simulink model "fcsystemBechmarkold"  (R2016a)
settings: Solver=FixedStepAuto  SolverMode=MultiTasking  StartTime=0.0  StopTime=30.0  FixedStep=0.0001  MaxStep=0.0001  RelTol=1e-5
InitFcn:
  | fcsmain;
values from neighbouring files (symbols this model uses):
  C = ss1.C    [MVE.m]
  G = ss1.A    [MVE.m]
  H = ss1.B    [MVE.m]
  K1 = Ktemp(1)    [MVE.m]
  K2 = Ktemp(2:end)    [MVE.m]
  Ke = acker(G',C',P)'    [MVE.m]
  Ts = 0.1    [MVE.m]
undefined symbols (not defined in the file or in its folder): alliedsignaleff, beta0, beta1, beta2, cm_kt, cm_kv, cm_maxtorque, cm_R, Cp, cp_inertia, dc, faradays, fc_activearea, fc_anode_volume, fc_cathode_volume, fc_inlet_flow_constant, fc_numberofcells, fc_outlet_flow_constant, fcx0, gamma, hydrogengasconstant, hydrogenmolarmass, im_volume, membranedrydensity, membranedryeqvweight, membranethickness, nitrogengasconstant, nitrogenmolarmass, om_At, om_Cd, om_outlet_choke_pr, om_volume, oxygengasconstant, oxygenmolarmass, phimax0, phimax1, phimax2, phimax3, phimax4, psimax0, psimax1, psimax2, psimax3, psimax4, psimax5, R, rho, Ta, universalgasconstant, vaporgasconstant, vapormolarmass
libraries: simulink x1
(part 1 of 3)
settings Model: ExtModeTrigMode=oneshot  ExtModeArmWhenConnect=off  Creator=Jay Tawee Pukrushpan  LastModifiedBy=luisd
settings DataIOCC: SaveFinalState=on  SaveFormat=Array  SignalLoggingSaveFormat=ModelDataLogs  SignalLoggingName=sigsOut
settings OptimizationCC: BooleanDataType=off
settings DebuggingCC: SaveWithParameterizedLinksMsg=none  UnderspecifiedInitializationDetection=Classic  MergeDetectMultiDrivingBlocksExec=none  SignalResolutionControl=TryResolveAllWithWarning  MultiTaskDSMMsg=warning  MultiTaskCondExecSysMsg=none  FcnCallInpInsideContextMsg=UseLocalSettings  AllowSymbolicDim=off  StateNameClashWarn=warning
settings HardwareCC: ProdBitPerPointer=32  ProdLargestAtomicFloat=None  ProdIntDivRoundTo=Undefined  ProdEndianess=Unspecified  ProdWordSize=32  ProdHWDeviceType=32-bit Generic  TargetUnknown=on
settings ModelReferenceCC: PropagateSignalLabelsOutOfModel=off
settings GRTTargetCC: CombineOutputUpdateFcns=off  GRTInterface=on
settings ConfigComp: CovModelRefEnable=Off  CovSFcnEnable=off

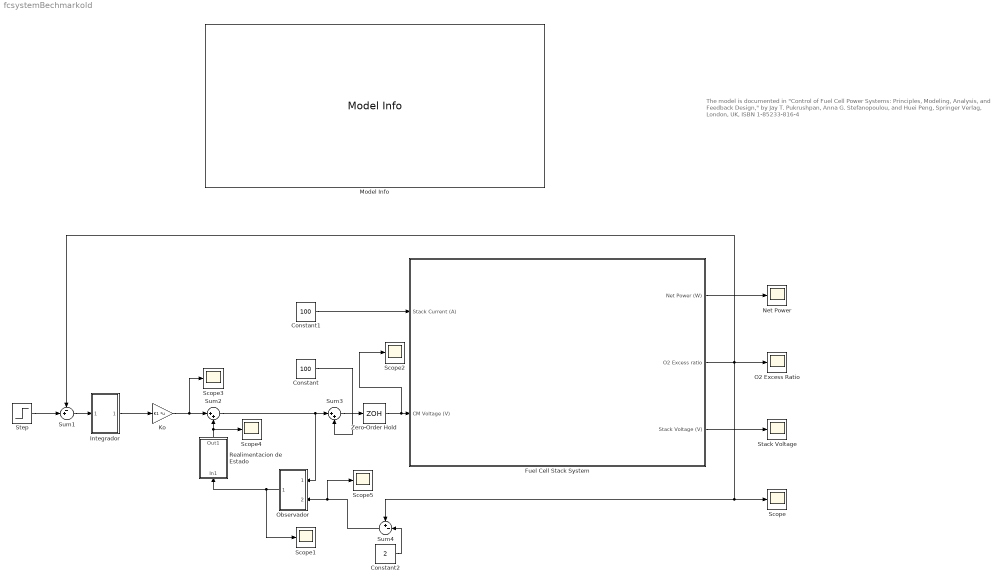
== system fcsystemBechmarkold ==
  note: The model is documented in
      | "Control of Fuel Cell Power Systems: Principles, Modeling, Analysis, and Feedback Design,"
      | by  Jay T. Pukrushpan, Anna G. Stefanopoulou, and Huei Peng,  Springer Verlag,
      | London, UK, ISBN 1-85233-816-4
  Constant : Constant  Value=100
  Constant1 : Constant  Value=100
  Constant2 : Constant  Value=2
  Fuel Cell Stack System : Subsystem
      mask Display:
      | image('Stack.jpg')
      | port_label('input', 1, 'corriente carga')
      | port_label('input', 2, 'tension compresor')
      | port_label('output', 1, 'potencia salida')
      | port_label('output', 2, 'exceso de oxigeno')
      | port_label('output', 3, 'tension de la pila')
  Integrador : Subsystem
  Ko : Gain  Gain=K1  Multiplication=Matrix(K*u)
  Model Info : simulink/Model-Wide Utilities/Model Info  Frame=on  DisplayStringWithTags=|  HorizontalTextAlignment=Left  LeftAlignmentValue=0.02  SourceBlockDiagram=fcsystemBechmark  TagMaxNumber=20
      | COPYRIGHT  © 2002 
      | THE REGENTS OF THE UNIVERSITY OF MICHIGAN
      | ALL RIGHTS RESERVED
      |       
      | PERMISSION IS GRANTED TO USE, COPY, CREATE DERIVATIVE WORKS AND REDISTRIBUTE THIS SOFTWARE AND SUCH 
      | DERIVATIVE WORKS FOR NONCOMMERCIAL EDUCATION AND RESEARCH PURPOSES, SO LONG AS NO FEE IS CHARGED, AND 
      | SO LONG AS THE COPYRIGHT NOTICE ABOVE, THIS GRANT OF PERMISSION, AND THE DISCLAIMER BELOW APPEAR IN ALL 
      | COPIES MADE; AND SO LONG AS THE NAME OF THE UNIVERSITY OF MICHIGAN IS NOT USED IN ANY ADVERTISING OR PUBLICITY 
      | PERTAINING TO THE USE OR DISTRIBUTION OF THIS SOFTWARE WITHOUT SPECIFIC, WRITTEN PRIOR AUTHORIZATION.
      |     
      | THIS USE OF THIS SOFTWARE REQUIRES SIMULINK, A LICENSED PRODUCT OF THE MATHWORKS, INC.  THE SOFTWARE 
      | USER IS SOLELY RESOPNSIBLE FOR OBTAINTING AN APPROPRIATE LICENSE FOR SIMULINK.  NO LICENSE TO SIMULINK 
      | IS GRANTED, INFERRED OR IMPLIED BY THE DISTRIBUTION OF THIS SOFTWARE.
      |     
      | THIS SOFTWARE IS PROVIDED AS IS, WITHOUT REPRESENTATION AS TO ITS FITNESS FOR ANY PURPOSE, AND WITHOUT 
      | WARRANTY OF ANY KIND, EITHER EXPRESS OR IMPLIED, INCLUDING WITHOUT LIMITATION THE IMPLIED WARRANTIES OF 
      | MERCHANTABILITY AND FITNESS FOR A PARTICULAR PURPOSE. THE REGENTS OF THE UNIVERSITY OF MICHIGAN SHALL NOT 
      | BE LIABLE FOR ANY DAMAGES, INCLUDING SPECIAL, INDIRECT, INCIDENTAL, OR CONSEQUENTIAL DAMAGES, WITH RESPECT
      | TO ANY CLAIM ARISING OUT OF OR IN CONNECTION WITH THE USE OF THE SOFTWARE, EVEN IF IT HAS BEEN OR IS HEREAFTER 
      | ADVISED OF THE POSSIBILITY OF SUCH DAMAGES.
  Net Power : Scope
  O2 Excess Ratio : Scope
  Observador : Subsystem
  Realimentacion de Estado : Subsystem
  Scope{,1..5} (6 alike) : Scope
  Stack Voltage : Scope
  Step : Step  Time=0  Before=2  After=2  SampleTime=Ts
  Sum1 : Sum  Inputs=-+|
  Sum2 : Sum  Inputs=|++
  Sum3 : Sum  Inputs=|++
  Sum4 : Sum  Inputs=+-|
  Zero-Order Hold : ZeroOrderHold  SampleTime=Ts
  wires:
  Sum2/1 -> Sum3/1, Observador/1(In1)
  Fuel Cell Stack System/1(Net Power (W)) -> Net Power/1
  Fuel Cell Stack System/3(Stack Voltage (V)) -> Stack Voltage/1
  Ko/1 -> Scope3/1, Sum2/1
  Realimentacion de Estado/1(Out1) -> Scope4/1, Sum2/2
  Observador/1(Out1) -> Scope1/1, Realimentacion de Estado/1(In1)
  Integrador/1(Out1) -> Ko/1
  Sum1/1 -> Integrador/1(In1)
  Step/1 -> Sum1/2
  Fuel Cell Stack System/2(O2 Excess ratio) -> Sum1/1, Sum4/1, Scope/1, O2 Excess Ratio/1
  Zero-Order Hold/1 -> Scope2/1, Fuel Cell Stack System/2(CM Voltage (V))
  Sum3/1 -> Zero-Order Hold/1
  Constant/1 -> Sum3/2
  Constant2/1 -> Sum4/2
  Sum4/1 -> Scope5/1, Observador/2(In2)
  Constant1/1 -> Fuel Cell Stack System/1(Stack Current (A))

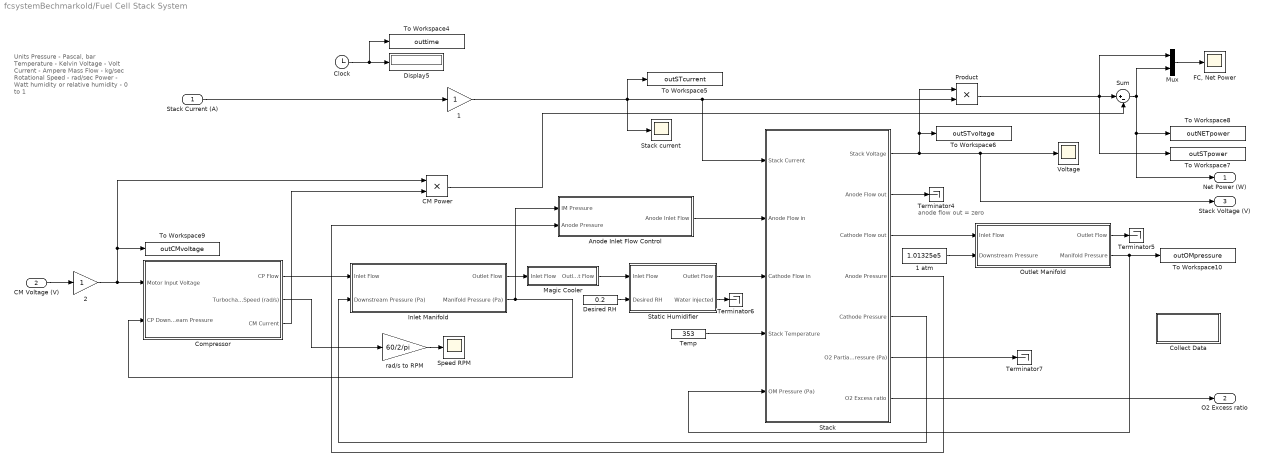
== system fcsystemBechmarkold/Fuel Cell Stack System ==
  note: Units
      | Pressure - Pascal, bar
      | Temperature - Kelvin
      | Voltage - Volt
      | Current - Ampere
      | Mass Flow - kg/sec
      | Rotational Speed - rad/sec
      | Power - Watt
      | humidity or relative humidity - 0 to 1
  note: anode flow out = zero
  Stack Current (A) : Inport
  CM Voltage (V) : Inport  Port=2
  " Outlet Manifold" : Subsystem
  1 : Gain  SaturateOnIntegerOverflow=on  OutDataTypeStr=Inherit: Same as input  ParamDataTypeStr=Inherit: Same as input
  1 atm : Constant  Value=1.01325e5
  2 : Gain  SaturateOnIntegerOverflow=on  OutDataTypeStr=Inherit: Same as input  ParamDataTypeStr=Inherit: Same as input
  Anode Inlet Flow Control : Subsystem
  CM Power : Product  SaturateOnIntegerOverflow=on  InputSameDT=on  OutDataTypeStr=Inherit: Same as first input
  Clock : Clock
  Collect Data : Subsystem
  Compressor : Subsystem
  Desired RH : Constant  Value=0.2
  Display5 : Display
  "FC, Net Power" : Scope
  Inlet Manifold : Subsystem
  Magic Cooler : Subsystem
  Mux : Mux  Inputs=2
  Product : Product  SaturateOnIntegerOverflow=on  InputSameDT=on  OutDataTypeStr=Inherit: Same as first input
  Speed RPM : Scope
  Stack : Subsystem
  Stack current : Scope
  Static Humidifier : Subsystem
  Sum : Sum  Inputs=|+-  SaturateOnIntegerOverflow=on  InputSameDT=on  OutDataTypeStr=Inherit: Same as first input
  Temp : Constant  Value=353
  Terminator{4..7} (4 alike) : Terminator
  To Workspace10 : ToWorkspace  VariableName=outOMpressure  SampleTime=-1
  To Workspace4 : ToWorkspace  VariableName=outtime  SampleTime=-1
  To Workspace5 : ToWorkspace  VariableName=outSTcurrent  SampleTime=-1
  To Workspace6 : ToWorkspace  VariableName=outSTvoltage  SampleTime=-1
  To Workspace7 : ToWorkspace  VariableName=outSTpower  SampleTime=-1
  To Workspace8 : ToWorkspace  VariableName=outNETpower  SampleTime=-1
  To Workspace9 : ToWorkspace  VariableName=outCMvoltage  SampleTime=-1
  Voltage : Scope
  rad/s to RPM : Gain  Gain=60/2/pi  SaturateOnIntegerOverflow=on  OutDataTypeStr=Inherit: Same as input  ParamDataTypeStr=Inherit: Same as input
  Net Power (W) : Outport
  O2 Excess ratio : Outport  Port=2
  Stack Voltage (V) : Outport  Port=3
  wires:
  Temp/1 -> Stack/4(Stack Temperature)
  Anode Inlet Flow Control/1(Anode Inlet Flow) -> Stack/2(Anode Flow in)
  rad/s to RPM/1 -> Speed RPM/1
  Inlet Manifold/1(Outlet Flow) -> Magic Cooler/1(Inlet Flow)
  1/1 -> Stack/1(Stack Current), Product/2, To Workspace5/1, Stack current/1
  Compressor/1(CP Flow) -> Inlet Manifold/1(Inlet Flow)
  Compressor/2(Turbocharger Speed (rad/s)) -> rad/s to RPM/1
  Magic Cooler/1(Outlet Flow) -> Static Humidifier/1(Inlet Flow)
  Desired RH/1 -> Static Humidifier/2(Desired RH)
  Stack/2(Anode Flow out) -> Terminator4/1
  " Outlet Manifold"/1(Outlet Flow) -> Terminator5/1
  Stack/4(Anode Pressure) -> Anode Inlet Flow Control/2(Anode Pressure)
  Product/1 -> To Workspace7/1, Mux/1, Sum/1
  Mux/1 -> "FC, Net Power"/1
  Sum/1 -> Mux/2, To Workspace8/1, Net Power (W)/1
  Stack/3(Cathode Flow out) -> " Outlet Manifold"/1(Inlet Flow)
  1 atm/1 -> " Outlet Manifold"/2(Downstream Pressure)
  " Outlet Manifold"/2(Manifold Pressure) -> To Workspace10/1, Stack/5(OM Pressure (Pa))
  Static Humidifier/2(Water injected) -> Terminator6/1
  Static Humidifier/1(Outlet Flow) -> Stack/3(Cathode Flow in)
  CM Power/1 -> Sum/2
  Clock/1 -> To Workspace4/1, Display5/1
  Compressor/3(CM Current) -> CM Power/2
  Stack/5(Cathode Pressure) -> Inlet Manifold/2(Downstream Pressure (Pa))
  Inlet Manifold/2(Manifold Pressure (Pa)) -> Anode Inlet Flow Control/1(IM Pressure), Compressor/2(CP Downstream Pressure)
  Stack/6(O2 Partial Pressure (Pa)) -> Terminator7/1
  CM Voltage (V)/1 -> 2/1
  Stack/7(O2 Excess ratio) -> O2 Excess ratio/1
  Stack/1(Stack Voltage) -> Product/1, To Workspace6/1, Stack Voltage (V)/1, Voltage/1
  2/1 -> Compressor/1(Motor Input Voltage), To Workspace9/1, CM Power/1
  Stack Current (A)/1 -> 1/1

== system fcsystemBechmarkold/Integrador ==
  In1 : Inport
  Delay : Delay  DelayLength=1  InitialCondition=0  SampleTime=Ts
  Sum1 : Sum  Inputs=|++
  Out1 : Outport
  wires:
  Sum1/1 -> Out1/1, Delay/1
  In1/1 -> Sum1/1
  Delay/1 -> Sum1/2

== system fcsystemBechmarkold/Observador ==
  In1 : Inport
  In2 : Inport  Port=2
  C : Gain  Gain=C  Multiplication=Matrix(K*u)
  Delay : Delay  DelayLength=1  InitialCondition=1  SampleTime=Ts
  G : Gain  Gain=G  Multiplication=Matrix(K*u)
  H : Gain  Gain=H  Multiplication=Matrix(K*u)
  Ke : Gain  Gain=Ke  Multiplication=Matrix(K*u)
  Sum1 : Sum  Inputs=-+|
  Sum3 : Sum  Inputs=|++
  Sum4 : Sum  Inputs=|++
  Out1 : Outport
  wires:
  In2/1 -> Sum1/2
  Ke/1 -> Sum4/2
  G/1 -> Sum3/2
  C/1 -> Sum1/1
  Delay/1 -> Out1/1, G/1, C/1
  Sum4/1 -> Sum3/1
  In1/1 -> H/1
  Sum3/1 -> Delay/1
  H/1 -> Sum4/1
  Sum1/1 -> Ke/1

== system fcsystemBechmarkold/Realimentacion de Estado ==
  In1 : Inport
  K : Gain  Gain=-K2  Multiplication=Matrix(K*u)
  Out1 : Outport
  wires:
  K/1 -> Out1/1
  In1/1 -> K/1

== system fcsystemBechmarkold/Fuel Cell Stack System/ Outlet Manifold ==
  Inlet Flow : Inport
  Downstream Pressure : Inport  Port=2
  1 - Total Mass Flow 2 - Temperature 3 - Pressure 4 - Relative Humidity 5 - Oxygen Mole Fraction (in Dry Air) : Demux  Outputs=5
  1 - Total Mass Flow 2 - Temperature 3 - Pressure 4 - Relative Humidity 5 - Oxygen Mole Fraction (in Dry Air)1 : Mux  Inputs=5
  Gain1 : Gain  Gain=R  SaturateOnIntegerOverflow=on  OutDataTypeStr=Inherit: Same as input  ParamDataTypeStr=Inherit: Same as input
  Gain2 : Gain  Gain=1/om_volume  SaturateOnIntegerOverflow=on  OutDataTypeStr=Inherit: Same as input  ParamDataTypeStr=Inherit: Same as input
  Initial P_om : Constant  Value=fcx0(8)
  Nonlinear Nozzle : Subsystem
  P_om Integrator : Integrator  InitialConditionSource=external
  Product : Product  SaturateOnIntegerOverflow=on  InputSameDT=on  OutDataTypeStr=Inherit: Same as first input
  Sum1 : Sum  Inputs=|+-  SaturateOnIntegerOverflow=on  InputSameDT=on  OutDataTypeStr=Inherit: Same as first input
  Terminator7 : Terminator
  Outlet Flow : Outport
  Manifold Pressure : Outport  Port=2
  tag scope: P_om=global
  wires:
  Downstream Pressure/1 -> Nonlinear Nozzle/2(Atmospheric Pressure)
  1 - Total Mass Flow 2 - Temperature 3 - Pressure 4 - Relative Humidity 5 - Oxygen Mole Fraction (in Dry Air)/5 -> 1 - Total Mass Flow 2 - Temperature 3 - Pressure 4 - Relative Humidity 5 - Oxygen Mole Fraction (in Dry Air)1/5
  1 - Total Mass Flow 2 - Temperature 3 - Pressure 4 - Relative Humidity 5 - Oxygen Mole Fraction (in Dry Air)/4 -> 1 - Total Mass Flow 2 - Temperature 3 - Pressure 4 - Relative Humidity 5 - Oxygen Mole Fraction (in Dry Air)1/4
  Nonlinear Nozzle/1(Mass Air Flow) -> 1 - Total Mass Flow 2 - Temperature 3 - Pressure 4 - Relative Humidity 5 - Oxygen Mole Fraction (in Dry Air)1/1, Sum1/2
  1 - Total Mass Flow 2 - Temperature 3 - Pressure 4 - Relative Humidity 5 - Oxygen Mole Fraction (in Dry Air)1/1 -> Outlet Flow/1
  1 - Total Mass Flow 2 - Temperature 3 - Pressure 4 - Relative Humidity 5 - Oxygen Mole Fraction (in Dry Air)/3 -> Terminator7/1
  1 - Total Mass Flow 2 - Temperature 3 - Pressure 4 - Relative Humidity 5 - Oxygen Mole Fraction (in Dry Air)/1 -> Sum1/1
  Inlet Flow/1 -> 1 - Total Mass Flow 2 - Temperature 3 - Pressure 4 - Relative Humidity 5 - Oxygen Mole Fraction (in Dry Air)/1
  1 - Total Mass Flow 2 - Temperature 3 - Pressure 4 - Relative Humidity 5 - Oxygen Mole Fraction (in Dry Air)/2 -> 1 - Total Mass Flow 2 - Temperature 3 - Pressure 4 - Relative Humidity 5 - Oxygen Mole Fraction (in Dry Air)1/2, Nonlinear Nozzle/3(Flow Temp), Gain1/1
  Gain1/1 -> Gain2/1
  Sum1/1 -> Product/1
  Gain2/1 -> Product/2
  P_om Integrator/1 -> 1 - Total Mass Flow 2 - Temperature 3 - Pressure 4 - Relative Humidity 5 - Oxygen Mole Fraction (in Dry Air)1/3, Manifold Pressure/1, [P_om], Nonlinear Nozzle/1(Manifold Pressure)
  Product/1 -> P_om Integrator/1
  Initial P_om/1 -> P_om Integrator/2

== system fcsystemBechmarkold/Fuel Cell Stack System/Anode Inlet Flow Control ==
  IM Pressure : Inport
  Anode Pressure : Inport  Port=2
  1 - Total Mass Flow 2 - Temperature 3 - Pressure 4 - Relative Humidity : Mux
  Gain : Gain  SaturateOnIntegerOverflow=on  OutDataTypeStr=Inherit: Same as input  ParamDataTypeStr=Inherit: Same as input
  Gain1 : Gain  Gain=2.1e-6  SaturateOnIntegerOverflow=on  OutDataTypeStr=Inherit: Same as input  ParamDataTypeStr=Inherit: Same as input
  RH : Constant  Value=0.4
  Sum : Sum  Inputs=|+-  SaturateOnIntegerOverflow=on  InputSameDT=on  OutDataTypeStr=Inherit: Same as first input
  Temp : Constant  Value=353
  pim to pca map : Fcn  Expr=(0.00092256030284*u+2.84870103138421)*1e3
  Anode Inlet Flow : Outport
  wires:
  Anode Pressure/1 -> 1 - Total Mass Flow 2 - Temperature 3 - Pressure 4 - Relative Humidity/3, Sum/2
  pim to pca map/1 -> Sum/1
  IM Pressure/1 -> pim to pca map/1
  Gain1/1 -> Gain/1
  Sum/1 -> Gain1/1
  RH/1 -> 1 - Total Mass Flow 2 - Temperature 3 - Pressure 4 - Relative Humidity/4
  Gain/1 -> 1 - Total Mass Flow 2 - Temperature 3 - Pressure 4 - Relative Humidity/1
  Temp/1 -> 1 - Total Mass Flow 2 - Temperature 3 - Pressure 4 - Relative Humidity/2
  1 - Total Mass Flow 2 - Temperature 3 - Pressure 4 - Relative Humidity/1 -> Anode Inlet Flow/1

== system fcsystemBechmarkold/Fuel Cell Stack System/Collect Data ==
  Mux : Mux  Inputs=9
  To Workspace : ToWorkspace  VariableName=outstates  SampleTime=-1
  wires:
  Mux/1 -> To Workspace/1
  [mw_ca] -> Mux/9
  [P_om] -> Mux/8
  [mw_an] -> Mux/7
  [m_im] -> Mux/6
  [P_im] -> Mux/5
  [w_cp] -> Mux/4
  [mN2] -> Mux/3
  [mH2] -> Mux/2
  [mO2] -> Mux/1

== system fcsystemBechmarkold/Fuel Cell Stack System/Compressor ==
  Motor Input Voltage : Inport
  CP Downstream Pressure : Inport  Port=2
  Compressor : Subsystem
  Constant : Constant  Value=0
  Constant1 : Constant  Value=0.5
  Static Motor : Subsystem
  To Workspace1 : ToWorkspace  VariableName=outCPspeed  SampleTime=-1
  To Workspace3 : ToWorkspace  VariableName=outCPpower  SampleTime=-1
  To Workspace4 : ToWorkspace  VariableName=outCMpower  SampleTime=-1
  Turbocharger Inertia : Subsystem
  CP Flow : Outport
  Turbocharger Speed (rad/s) : Outport  Port=2
  CM Current : Outport  Port=3
  wires:
  Static Motor/2(Motor Current) -> CM Current/1
  Motor Input Voltage/1 -> Static Motor/1(Input Voltage)
  Static Motor/1(Motor Power) -> To Workspace4/1, Turbocharger Inertia/1(Motor Power)
  Compressor/2(Power) -> To Workspace3/1, Turbocharger Inertia/2(Compressor Power)
  Constant1/1 -> Compressor/3(Inlet Humidity)
  Turbocharger Inertia/1(Speed) -> To Workspace1/1, Turbocharger Speed (rad/s)/1, Compressor/2(Speed), Static Motor/2(Motor Speed (rad/s))
  CP Downstream Pressure/1 -> Compressor/1(Exit Pressure (Pa))
  Compressor/1(CP Flow) -> CP Flow/1
  Constant/1 -> Turbocharger Inertia/3(Turbine Power)

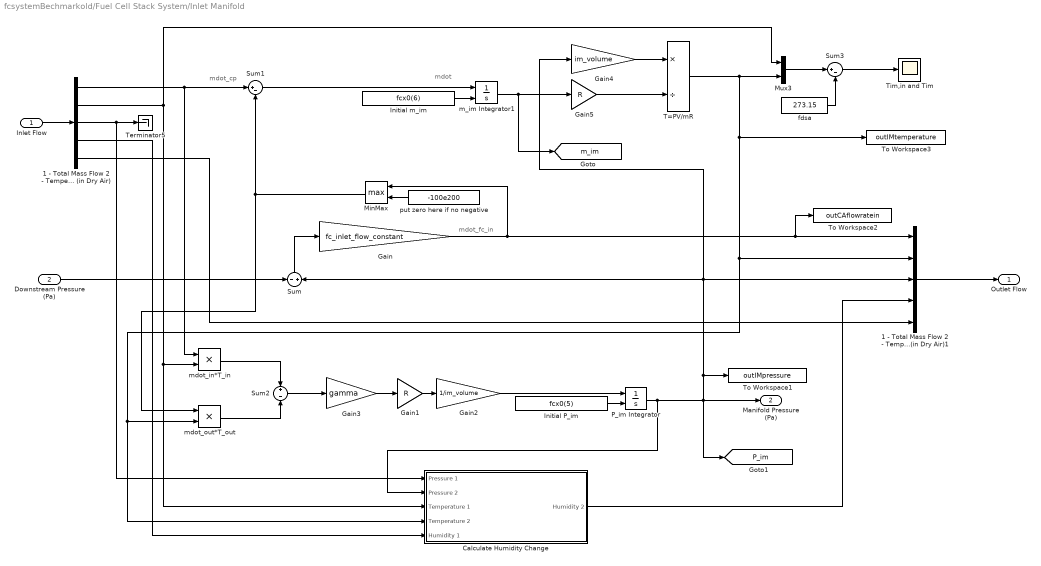
== system fcsystemBechmarkold/Fuel Cell Stack System/Inlet Manifold ==
  note: mdot_cp
  note: mdot_fc_in
  note: mdot
  Inlet Flow : Inport
  Downstream Pressure (Pa) : Inport  Port=2
  1 - Total Mass Flow 2 - Temperature 3 - Pressure 4 - Relative Humidity 5 - Oxygen Mole Fraction (in Dry Air) : Demux  Outputs=5
  1 - Total Mass Flow 2 - Temperature 3 - Pressure 4 - Relative Humidity 5 - Oxygen Mole Fraction (in Dry Air)1 : Mux  Inputs=5
  Calculate Humidity Change : Subsystem
  Gain : Gain  Gain=fc_inlet_flow_constant  SaturateOnIntegerOverflow=on  OutDataTypeStr=Inherit: Same as input  ParamDataTypeStr=Inherit: Same as input
  Gain1 : Gain  Gain=R  SaturateOnIntegerOverflow=on  OutDataTypeStr=Inherit: Same as input  ParamDataTypeStr=Inherit: Same as input
  Gain2 : Gain  Gain=1/im_volume  SaturateOnIntegerOverflow=on  OutDataTypeStr=Inherit: Same as input  ParamDataTypeStr=Inherit: Same as input
  Gain3 : Gain  Gain=gamma  SaturateOnIntegerOverflow=on  OutDataTypeStr=Inherit: Same as input  ParamDataTypeStr=Inherit: Same as input
  Gain4 : Gain  Gain=im_volume  SaturateOnIntegerOverflow=on  OutDataTypeStr=Inherit: Same as input  ParamDataTypeStr=Inherit: Same as input
  Gain5 : Gain  Gain=R  SaturateOnIntegerOverflow=on  OutDataTypeStr=Inherit: Same as input  ParamDataTypeStr=Inherit: Same as input
  Initial P_im : Constant  Value=fcx0(5)
  Initial m_im : Constant  Value=fcx0(6)
  MinMax : MinMax  Function=max  Inputs=2  SaturateOnIntegerOverflow=on  InputSameDT=on
  Mux3 : Mux  Inputs=2
  P_im Integrator : Integrator  InitialConditionSource=external
  Sum : Sum  Inputs=-|+  SaturateOnIntegerOverflow=on  InputSameDT=on  OutDataTypeStr=Inherit: Same as first input
  Sum1 : Sum  Inputs=|+-  SaturateOnIntegerOverflow=on  InputSameDT=on  OutDataTypeStr=Inherit: Same as first input
  Sum2 : Sum  Inputs=+-  SaturateOnIntegerOverflow=on  InputSameDT=on  OutDataTypeStr=Inherit: Same as first input
  Sum3 : Sum  Inputs=|+-  SaturateOnIntegerOverflow=on  InputSameDT=on  OutDataTypeStr=Inherit: Same as first input
  T=PV/mR : Product  Inputs=*/  SaturateOnIntegerOverflow=on  InputSameDT=on  OutDataTypeStr=Inherit: Same as first input
  Terminator5 : Terminator
  Tim,in and Tim : Scope
  To Workspace1 : ToWorkspace  VariableName=outIMpressure  SampleTime=-1
  To Workspace2 : ToWorkspace  VariableName=outCAflowratein  SampleTime=-1
  To Workspace3 : ToWorkspace  VariableName=outIMtemperature  SampleTime=-1
  fdsa : Constant  Value=273.15
  m_im Integrator1 : Integrator  InitialConditionSource=external
  mdot_in*T_in : Product  SaturateOnIntegerOverflow=on  InputSameDT=on  OutDataTypeStr=Inherit: Same as first input
  mdot_out*T_out : Product  SaturateOnIntegerOverflow=on  InputSameDT=on  OutDataTypeStr=Inherit: Same as first input
  put zero here if no negative : Constant  Value=-100e200
  Outlet Flow : Outport
  Manifold Pressure (Pa) : Outport  Port=2
  tag scope: P_im=global, m_im=global
  wires:
  Calculate Humidity Change/1(Humidity 2) -> 1 - Total Mass Flow 2 - Temperature 3 - Pressure 4 - Relative Humidity 5 - Oxygen Mole Fraction (in Dry Air)1/4
  1 - Total Mass Flow 2 - Temperature 3 - Pressure 4 - Relative Humidity 5 - Oxygen Mole Fraction (in Dry Air)/4 -> Calculate Humidity Change/5(Humidity 1)
  1 - Total Mass Flow 2 - Temperature 3 - Pressure 4 - Relative Humidity 5 - Oxygen Mole Fraction (in Dry Air)/3 -> Calculate Humidity Change/1(Pressure 1), Terminator5/1
  fdsa/1 -> Sum3/2
  Sum3/1 -> Tim,in and Tim/1
  Mux3/1 -> Sum3/1
  1 - Total Mass Flow 2 - Temperature 3 - Pressure 4 - Relative Humidity 5 - Oxygen Mole Fraction (in Dry Air)/2 -> Calculate Humidity Change/3(Temperature 1), mdot_in*T_in/2, Mux3/1
  T=PV/mR/1 -> To Workspace3/1, Calculate Humidity Change/4(Temperature 2), mdot_out*T_out/2, 1 - Total Mass Flow 2 - Temperature 3 - Pressure 4 - Relative Humidity 5 - Oxygen Mole Fraction (in Dry Air)1/2, Mux3/2
  Gain/1 -> To Workspace2/1, 1 - Total Mass Flow 2 - Temperature 3 - Pressure 4 - Relative Humidity 5 - Oxygen Mole Fraction (in Dry Air)1/1, MinMax/1
  Inlet Flow/1 -> 1 - Total Mass Flow 2 - Temperature 3 - Pressure 4 - Relative Humidity 5 - Oxygen Mole Fraction (in Dry Air)/1
  Downstream Pressure (Pa)/1 -> Sum/1
  Sum/1 -> Gain/1
  1 - Total Mass Flow 2 - Temperature 3 - Pressure 4 - Relative Humidity 5 - Oxygen Mole Fraction (in Dry Air)1/1 -> Outlet Flow/1
  Initial m_im/1 -> m_im Integrator1/2
  Sum1/1 -> m_im Integrator1/1
  put zero here if no negative/1 -> MinMax/2
  1 - Total Mass Flow 2 - Temperature 3 - Pressure 4 - Relative Humidity 5 - Oxygen Mole Fraction (in Dry Air)/1 -> Sum1/1, mdot_in*T_in/1
  MinMax/1 -> Sum1/2, mdot_out*T_out/1
  mdot_in*T_in/1 -> Sum2/1
  mdot_out*T_out/1 -> Sum2/2
  Gain1/1 -> Gain2/1
  Gain3/1 -> Gain1/1
  Sum2/1 -> Gain3/1
  Gain2/1 -> P_im Integrator/1
  Initial P_im/1 -> P_im Integrator/2
  Gain4/1 -> T=PV/mR/1
  Gain5/1 -> T=PV/mR/2
  1 - Total Mass Flow 2 - Temperature 3 - Pressure 4 - Relative Humidity 5 - Oxygen Mole Fraction (in Dry Air)/5 -> 1 - Total Mass Flow 2 - Temperature 3 - Pressure 4 - Relative Humidity 5 - Oxygen Mole Fraction (in Dry Air)1/5
  m_im Integrator1/1 -> Gain5/1, [m_im]
  P_im Integrator/1 -> Calculate Humidity Change/2(Pressure 2), Manifold Pressure (Pa)/1, To Workspace1/1, 1 - Total Mass Flow 2 - Temperature 3 - Pressure 4 - Relative Humidity 5 - Oxygen Mole Fraction (in Dry Air)1/3, Sum/2, Gain4/1, [P_im]

== system fcsystemBechmarkold/Fuel Cell Stack System/Magic Cooler ==
  Inlet Flow : Inport
  1 - Total Mass Flow 2 - Temperature 3 - Pressure 4 - Relative Humidity 5 - Oxygen Mole Fraction (in Dry Air) : Demux  Outputs=5
  1 - Total Mass Flow 2 - Temperature 3 - Pressure 4 - Relative Humidity 5 - Oxygen Mole Fraction (in Dry Air)1 : Mux  Inputs=5
  Assume magic cooler : Constant  Value=353
  Calculate Humidity Change : Subsystem
  Outlet Flow : Outport
  wires:
  Calculate Humidity Change/1(Humidity 2) -> 1 - Total Mass Flow 2 - Temperature 3 - Pressure 4 - Relative Humidity 5 - Oxygen Mole Fraction (in Dry Air)1/4
  1 - Total Mass Flow 2 - Temperature 3 - Pressure 4 - Relative Humidity 5 - Oxygen Mole Fraction (in Dry Air)/4 -> Calculate Humidity Change/5(Humidity 1)
  Assume magic cooler/1 -> Calculate Humidity Change/4(Temperature 2), 1 - Total Mass Flow 2 - Temperature 3 - Pressure 4 - Relative Humidity 5 - Oxygen Mole Fraction (in Dry Air)1/2
  1 - Total Mass Flow 2 - Temperature 3 - Pressure 4 - Relative Humidity 5 - Oxygen Mole Fraction (in Dry Air)/2 -> Calculate Humidity Change/3(Temperature 1)
  1 - Total Mass Flow 2 - Temperature 3 - Pressure 4 - Relative Humidity 5 - Oxygen Mole Fraction (in Dry Air)/3 -> Calculate Humidity Change/1(Pressure 1), Calculate Humidity Change/2(Pressure 2), 1 - Total Mass Flow 2 - Temperature 3 - Pressure 4 - Relative Humidity 5 - Oxygen Mole Fraction (in Dry Air)1/3
  1 - Total Mass Flow 2 - Temperature 3 - Pressure 4 - Relative Humidity 5 - Oxygen Mole Fraction (in Dry Air)/5 -> 1 - Total Mass Flow 2 - Temperature 3 - Pressure 4 - Relative Humidity 5 - Oxygen Mole Fraction (in Dry Air)1/5
  1 - Total Mass Flow 2 - Temperature 3 - Pressure 4 - Relative Humidity 5 - Oxygen Mole Fraction (in Dry Air)1/1 -> Outlet Flow/1
  1 - Total Mass Flow 2 - Temperature 3 - Pressure 4 - Relative Humidity 5 - Oxygen Mole Fraction (in Dry Air)/1 -> 1 - Total Mass Flow 2 - Temperature 3 - Pressure 4 - Relative Humidity 5 - Oxygen Mole Fraction (in Dry Air)1/1
  Inlet Flow/1 -> 1 - Total Mass Flow 2 - Temperature 3 - Pressure 4 - Relative Humidity 5 - Oxygen Mole Fraction (in Dry Air)/1

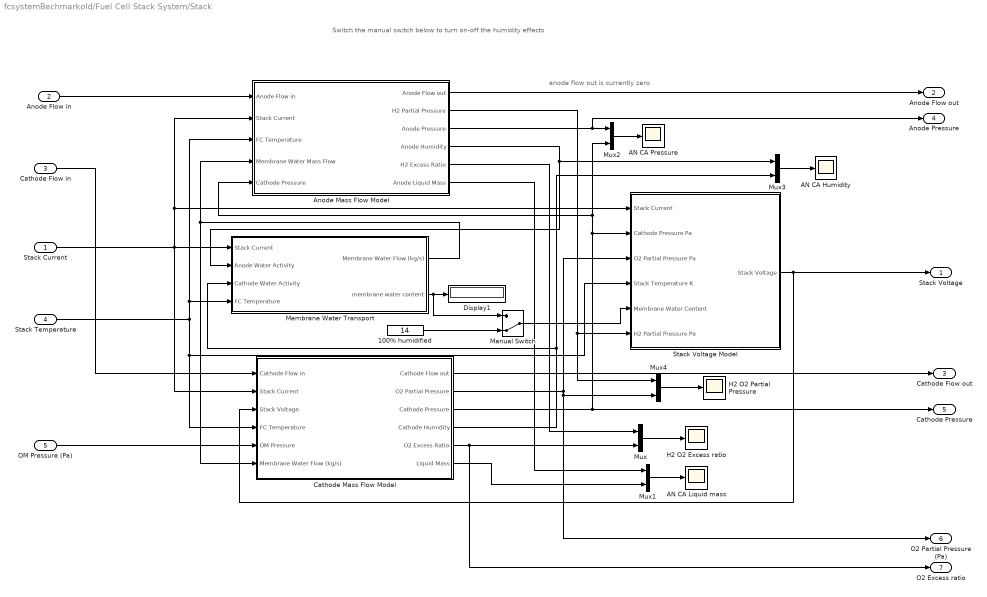
== system fcsystemBechmarkold/Fuel Cell Stack System/Stack ==
  note: anode flow out is currently zero
  note: Switch the manual switch below to turn on-off the humidity effects
  Stack Current : Inport
  Anode Flow in : Inport  Port=2
  Cathode Flow in : Inport  Port=3
  Stack Temperature : Inport  Port=4
  OM Pressure (Pa) : Inport  Port=5
  100% humidified : Constant  Value=14
  AN CA Humidity : Scope
  AN CA Liquid mass : Scope
  AN CA Pressure : Scope
  Anode Mass Flow Model : Subsystem
  Cathode Mass Flow Model : Subsystem
  Display1 : Display
  H2 O2 Excess ratio : Scope
  H2 O2 Partial Pressure : Scope
  Manual Switch : ManualSwitch  CurrentSetting=0
  Membrane Water Transport : Subsystem
  Mux{,1..4} (5 alike) : Mux  Inputs=2
  Stack Voltage Model : Subsystem
  Stack Voltage : Outport
  Anode Flow out : Outport  Port=2
  Cathode Flow out : Outport  Port=3
  Anode Pressure : Outport  Port=4
  Cathode Pressure : Outport  Port=5
  O2 Partial Pressure (Pa) : Outport  Port=6
  O2 Excess ratio : Outport  Port=7
  wires:
  Membrane Water Transport/2(membrane water content) -> Display1/1, Manual Switch/1
  Manual Switch/1 -> Stack Voltage Model/5(Membrane Water Content)
  100% humidified/1 -> Manual Switch/2
  Cathode Mass Flow Model/2(O2 Partial Pressure) -> O2 Partial Pressure (Pa)/1, Mux4/2, Stack Voltage Model/3(O2 Partial Pressure Pa)
  Anode Mass Flow Model/2(H2 Partial Pressure) -> Mux4/1, Stack Voltage Model/6(H2 Partial Pressure Pa)
  Mux4/1 -> H2 O2 Partial Pressure/1
  Cathode Mass Flow Model/5(O2 Excess Ratio) -> Mux/2, O2 Excess ratio/1
  Cathode Mass Flow Model/4(Cathode Humidity) -> Membrane Water Transport/3(Cathode Water Activity), Mux3/2
  Mux3/1 -> AN CA Humidity/1
  Anode Mass Flow Model/4(Anode Humidity) -> Membrane Water Transport/2(Anode Water Activity), Mux3/1
  Anode Mass Flow Model/6(Anode Liquid Mass) -> Mux1/1
  Stack Voltage Model/1(Stack Voltage) -> Cathode Mass Flow Model/3(Stack Voltage), Stack Voltage/1
  Mux1/1 -> AN CA Liquid mass/1
  Mux/1 -> H2 O2 Excess ratio/1
  Anode Mass Flow Model/3(Anode Pressure) -> Mux2/1, Anode Pressure/1
  Cathode Mass Flow Model/3(Cathode Pressure) -> Cathode Pressure/1, Stack Voltage Model/2(Cathode Pressure Pa), Anode Mass Flow Model/5(Cathode Pressure), Mux2/2
  Mux2/1 -> AN CA Pressure/1
  Cathode Mass Flow Model/6(Liquid Mass) -> Mux1/2
  Anode Mass Flow Model/5(H2 Excess Ratio) -> Mux/1
  Cathode Mass Flow Model/1(Cathode Flow out) -> Cathode Flow out/1
  Anode Mass Flow Model/1(Anode Flow out) -> Anode Flow out/1
  OM Pressure (Pa)/1 -> Cathode Mass Flow Model/5(OM Pressure)
  Stack Temperature/1 -> Anode Mass Flow Model/3(FC Temperature), Membrane Water Transport/4(FC Temperature), Cathode Mass Flow Model/4(FC Temperature), Stack Voltage Model/4(Stack Temperature K)
  Stack Current/1 -> Membrane Water Transport/1(Stack Current), Cathode Mass Flow Model/2(Stack Current), Anode Mass Flow Model/2(Stack Current), Stack Voltage Model/1(Stack Current)
  Cathode Flow in/1 -> Cathode Mass Flow Model/1(Cathode Flow in)
  Anode Flow in/1 -> Anode Mass Flow Model/1(Anode Flow in)
  Membrane Water Transport/1(Membrane Water Flow (kg/s)) -> Anode Mass Flow Model/4(Membrane Water Mass Flow), Cathode Mass Flow Model/6(Membrane Water Flow (kg/s))

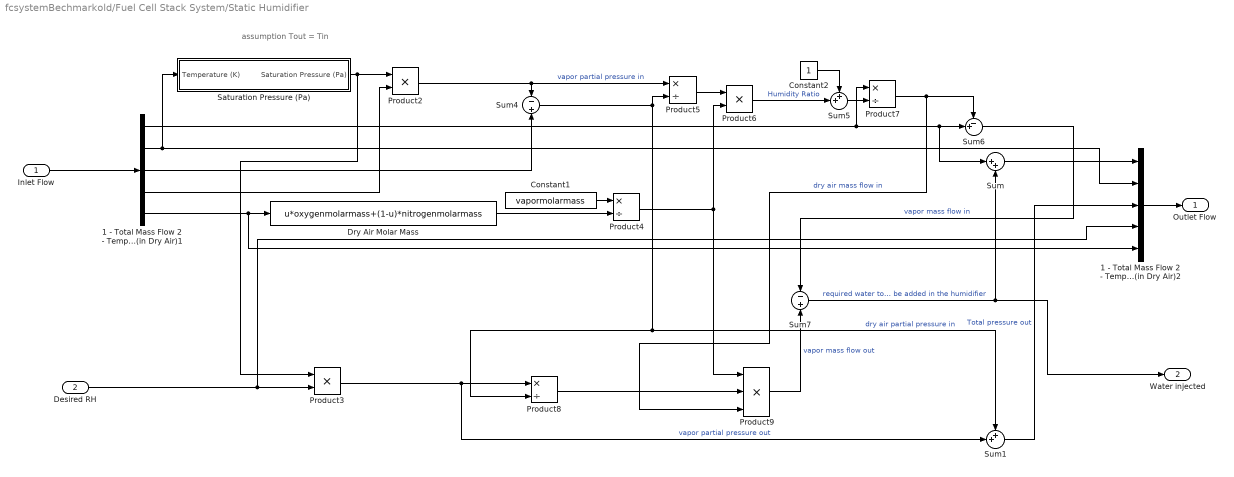
== system fcsystemBechmarkold/Fuel Cell Stack System/Static Humidifier ==
  note: assumption
      | Tout = Tin
  Inlet Flow : Inport
  Desired RH : Inport  Port=2
  1 - Total Mass Flow 2 - Temperature 3 - Pressure 4 - Relative Humidity 5 - Oxygen Mole Fraction (in Dry Air)1 : Demux  Outputs=5
  1 - Total Mass Flow 2 - Temperature 3 - Pressure 4 - Relative Humidity 5 - Oxygen Mole Fraction (in Dry Air)2 : Mux  Inputs=5
  Constant1 : Constant  Value=vapormolarmass
  Constant2 : Constant
  Dry Air Molar Mass : Fcn  Expr=u*oxygenmolarmass+(1-u)*nitrogenmolarmass
  Product2 : Product  SaturateOnIntegerOverflow=on  InputSameDT=on  OutDataTypeStr=Inherit: Same as first input
  Product3 : Product  SaturateOnIntegerOverflow=on  InputSameDT=on  OutDataTypeStr=Inherit: Same as first input
  Product{4..5,7..8} (4 alike) : Product  Inputs=*/  SaturateOnIntegerOverflow=on  InputSameDT=on  OutDataTypeStr=Inherit: Same as first input
  Product6 : Product  SaturateOnIntegerOverflow=on  InputSameDT=on  OutDataTypeStr=Inherit: Same as first input
  Product9 : Product  Inputs=3  SaturateOnIntegerOverflow=on  InputSameDT=on  OutDataTypeStr=Inherit: Same as first input
  Saturation Pressure (Pa) : Subsystem
  Sum : Sum  Inputs=|++  SaturateOnIntegerOverflow=on  InputSameDT=on  OutDataTypeStr=Inherit: Same as first input
  Sum1 : Sum  Inputs=++|  SaturateOnIntegerOverflow=on  InputSameDT=on  OutDataTypeStr=Inherit: Same as first input
  Sum4 : Sum  Inputs=-|+  SaturateOnIntegerOverflow=on  InputSameDT=on  OutDataTypeStr=Inherit: Same as first input
  Sum5 : Sum  Inputs=++|  SaturateOnIntegerOverflow=on  InputSameDT=on  OutDataTypeStr=Inherit: Same as first input
  Sum6 : Sum  Inputs=-+|  SaturateOnIntegerOverflow=on  InputSameDT=on  OutDataTypeStr=Inherit: Same as first input
  Sum7 : Sum  Inputs=-|+  SaturateOnIntegerOverflow=on  InputSameDT=on  OutDataTypeStr=Inherit: Same as first input
  Outlet Flow : Outport
  Water injected : Outport  Port=2
  wires:
  1 - Total Mass Flow 2 - Temperature 3 - Pressure 4 - Relative Humidity 5 - Oxygen Mole Fraction (in Dry Air)2/1 -> Outlet Flow/1
  Inlet Flow/1 -> 1 - Total Mass Flow 2 - Temperature 3 - Pressure 4 - Relative Humidity 5 - Oxygen Mole Fraction (in Dry Air)1/1
  1 - Total Mass Flow 2 - Temperature 3 - Pressure 4 - Relative Humidity 5 - Oxygen Mole Fraction (in Dry Air)1/4 -> Product2/2
  Dry Air Molar Mass/1 -> Product4/2
  Constant1/1 -> Product4/1
  1 - Total Mass Flow 2 - Temperature 3 - Pressure 4 - Relative Humidity 5 - Oxygen Mole Fraction (in Dry Air)1/2 -> Saturation Pressure (Pa)/1(Temperature (K)), 1 - Total Mass Flow 2 - Temperature 3 - Pressure 4 - Relative Humidity 5 - Oxygen Mole Fraction (in Dry Air)2/2
  Desired RH/1 -> Product3/2, 1 - Total Mass Flow 2 - Temperature 3 - Pressure 4 - Relative Humidity 5 - Oxygen Mole Fraction (in Dry Air)2/4
  Saturation Pressure (Pa)/1(Saturation Pressure (Pa)) -> Product2/1, Product3/1
  1 - Total Mass Flow 2 - Temperature 3 - Pressure 4 - Relative Humidity 5 - Oxygen Mole Fraction (in Dry Air)1/5 -> Dry Air Molar Mass/1, 1 - Total Mass Flow 2 - Temperature 3 - Pressure 4 - Relative Humidity 5 - Oxygen Mole Fraction (in Dry Air)2/5
  Product6/1 -> Sum5/2  "Humidity Ratio"
  Sum5/1 -> Product7/2
  Product5/1 -> Product6/1
  1 - Total Mass Flow 2 - Temperature 3 - Pressure 4 - Relative Humidity 5 - Oxygen Mole Fraction (in Dry Air)1/1 -> Product7/1, Sum6/2, Sum/1
  1 - Total Mass Flow 2 - Temperature 3 - Pressure 4 - Relative Humidity 5 - Oxygen Mole Fraction (in Dry Air)1/3 -> Sum4/2
  Constant2/1 -> Sum5/1
  Sum4/1 -> Product5/2, Sum1/1, Product8/2  "dry air partial pressure in"
  Product7/1 -> Product9/3, Sum6/1  "dry air mass flow in"
  Product4/1 -> Product9/1, Product6/2
  Sum/1 -> 1 - Total Mass Flow 2 - Temperature 3 - Pressure 4 - Relative Humidity 5 - Oxygen Mole Fraction (in Dry Air)2/1
  Sum1/1 -> 1 - Total Mass Flow 2 - Temperature 3 - Pressure 4 - Relative Humidity 5 - Oxygen Mole Fraction (in Dry Air)2/3  "Total pressure out"
  Sum6/1 -> Sum7/1  "vapor mass flow in"
  Product9/1 -> Sum7/2  "vapor mass flow out"
  Sum7/1 -> Water injected/1, Sum/2  "required water to be added in the humidifier"
  Product3/1 -> Product8/1, Sum1/2  "vapor partial pressure out"
  Product2/1 -> Sum4/1, Product5/1  "vapor partial pressure in"
  Product8/1 -> Product9/2

== system fcsystemBechmarkold/Fuel Cell Stack System/ Outlet Manifold/Nonlinear Nozzle ==
  Manifold Pressure : Inport
  Atmospheric Pressure : Inport  Port=2
  Flow Temp : Inport  Port=3
  1 - Upstream Pressure 2 - Downstream Pressure 3 - Temperature : Mux  Inputs=3
  1 - Upstream Pressure 2 - Temperature : Mux  Inputs=2
  Mass Flow Rate (choke) : Fcn  Expr=om_Cd*om_At*u[1]/sqrt(universalgasconstant*u[2])*sqrt(gamma)*(2/(gamma+1))^((gamma+1)/2/(gamma-1))
  Mass Flow Rate (sub critical) : Fcn  Expr=om_Cd*om_At*u[1]/sqrt(universalgasconstant*u[3])*(u[2]/u[1])^(1/gamma)*sqrt(2*gamma/(gamma-1)*(1-(u[2]/u[1])^((gamma-1)/gamma)))
  Product : Product  Inputs=*/  SaturateOnIntegerOverflow=on  InputSameDT=on  OutDataTypeStr=Inherit: Same as first input
  Switch > not choke < choke : Switch  Threshold=om_outlet_choke_pr  SaturateOnIntegerOverflow=on  InputSameDT=on
  Mass Air Flow : Outport
  wires:
  Product/1 -> Switch > not choke < choke/2
  Switch > not choke < choke/1 -> Mass Air Flow/1
  Manifold Pressure/1 -> Product/2, 1 - Upstream Pressure 2 - Temperature/1, 1 - Upstream Pressure 2 - Downstream Pressure 3 - Temperature/1
  Mass Flow Rate (choke)/1 -> Switch > not choke < choke/3
  Atmospheric Pressure/1 -> Product/1, 1 - Upstream Pressure 2 - Downstream Pressure 3 - Temperature/2
  1 - Upstream Pressure 2 - Downstream Pressure 3 - Temperature/1 -> Mass Flow Rate (sub critical)/1
  Mass Flow Rate (sub critical)/1 -> Switch > not choke < choke/1
  1 - Upstream Pressure 2 - Temperature/1 -> Mass Flow Rate (choke)/1
  Flow Temp/1 -> 1 - Upstream Pressure 2 - Temperature/2, 1 - Upstream Pressure 2 - Downstream Pressure 3 - Temperature/3

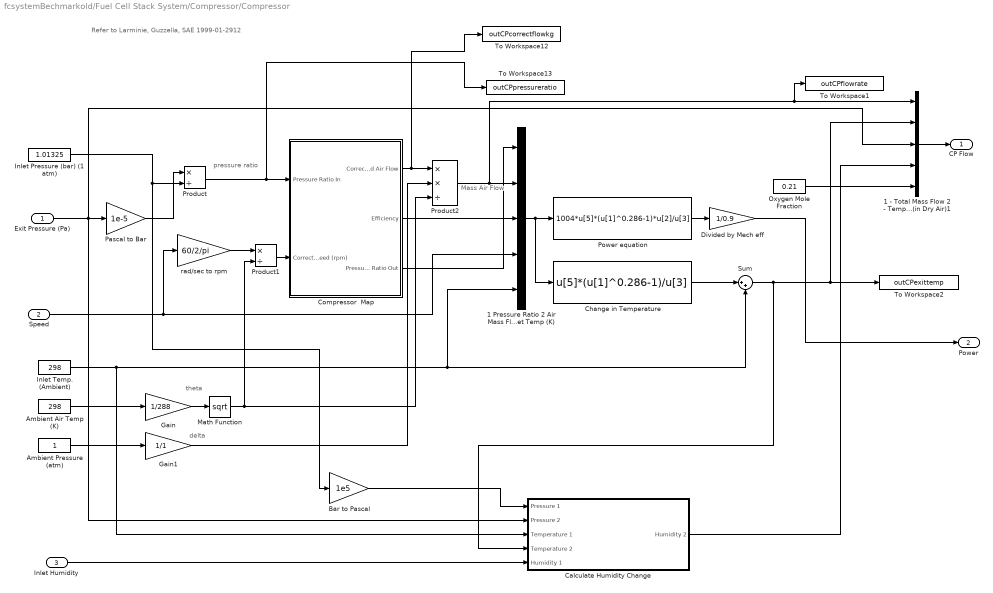
== system fcsystemBechmarkold/Fuel Cell Stack System/Compressor/Compressor ==
  note: Mass Air
      | Flow
  note: delta
  note: theta
  note: pressure
      | ratio
  note: Refer to Larminie, Guzzella, SAE 1999-01-2912
  Exit Pressure (Pa) : Inport
  Speed : Inport  Port=2
  Inlet Humidity : Inport  Port=3
  1 - Total Mass Flow 2 - Temperature 3 - Pressure 4 - Relative Humidity 5 - Oxygen Mole Fraction (in Dry Air)1 : Mux  Inputs=5
  1 Pressure Ratio 2 Air Mass Flow Rate 3 Efficiency 4 Speed (rad/sec) 5 Inlet Temp (K) : Mux  Inputs=5
  Ambient Air Temp (K) : Constant  Value=298
  Ambient Pressure (atm) : Constant
  Bar to Pascal : Gain  Gain=1e5  SaturateOnIntegerOverflow=on  OutDataTypeStr=Inherit: Same as input  ParamDataTypeStr=Inherit: Same as input
  Calculate Humidity Change : Subsystem
  Change in Temperature : Fcn  Expr=u[5]*(u[1]^0.286-1)/u[3]
  Compressor  Map : Subsystem
  Divided by Mech eff : Gain  Gain=1/0.9  SaturateOnIntegerOverflow=on  OutDataTypeStr=Inherit: Same as input  ParamDataTypeStr=Inherit: Same as input
  Gain : Gain  Gain=1/288  SaturateOnIntegerOverflow=on  OutDataTypeStr=Inherit: Same as input  ParamDataTypeStr=Inherit: Same as input
  Gain1 : Gain  Gain=1/1  SaturateOnIntegerOverflow=on  OutDataTypeStr=Inherit: Same as input  ParamDataTypeStr=Inherit: Same as input
  Inlet Pressure (bar) (1 atm) : Constant  Value=1.01325
  Inlet Temp. (Ambient) : Constant  Value=298
  Math Function : Math  Operator=sqrt  SaturateOnIntegerOverflow=on
  Oxygen Mole Fraction : Constant  Value=0.21
  Pascal to Bar : Gain  Gain=1e-5  SaturateOnIntegerOverflow=on  OutDataTypeStr=Inherit: Same as input  ParamDataTypeStr=Inherit: Same as input
  Power equation : Fcn  Expr=1004*u[5]*(u[1]^0.286-1)*u[2]/u[3]
  Product : Product  Inputs=*/  SaturateOnIntegerOverflow=on  InputSameDT=on  OutDataTypeStr=Inherit: Same as first input
  Product1 : Product  Inputs=*/  SaturateOnIntegerOverflow=on  InputSameDT=on  OutDataTypeStr=Inherit: Same as first input
  Product2 : Product  Inputs=**/  SaturateOnIntegerOverflow=on  InputSameDT=on  OutDataTypeStr=Inherit: Same as first input
  Sum : Sum  Inputs=|++  SaturateOnIntegerOverflow=on  InputSameDT=on  OutDataTypeStr=Inherit: Same as first input
  To Workspace1 : ToWorkspace  VariableName=outCPflowrate  SampleTime=-1
  To Workspace12 : ToWorkspace  VariableName=outCPcorrectflowkg  SampleTime=-1
  To Workspace13 : ToWorkspace  VariableName=outCPpressureratio  SampleTime=-1
  To Workspace2 : ToWorkspace  VariableName=outCPexittemp  SampleTime=-1
  rad/sec to rpm : Gain  Gain=60/2/pi  SaturateOnIntegerOverflow=on  OutDataTypeStr=Inherit: Same as input  ParamDataTypeStr=Inherit: Same as input
  CP Flow : Outport
  Power : Outport  Port=2
  wires:
  Oxygen Mole Fraction/1 -> 1 - Total Mass Flow 2 - Temperature 3 - Pressure 4 - Relative Humidity 5 - Oxygen Mole Fraction (in Dry Air)1/5
  Inlet Humidity/1 -> Calculate Humidity Change/5(Humidity 1)
  Bar to Pascal/1 -> Calculate Humidity Change/1(Pressure 1)
  Calculate Humidity Change/1(Humidity 2) -> 1 - Total Mass Flow 2 - Temperature 3 - Pressure 4 - Relative Humidity 5 - Oxygen Mole Fraction (in Dry Air)1/4
  Sum/1 -> Calculate Humidity Change/4(Temperature 2), To Workspace2/1, 1 - Total Mass Flow 2 - Temperature 3 - Pressure 4 - Relative Humidity 5 - Oxygen Mole Fraction (in Dry Air)1/2
  Inlet Temp. (Ambient)/1 -> Sum/2, 1 Pressure Ratio 2 Air Mass Flow Rate 3 Efficiency 4 Speed (rad/sec) 5 Inlet Temp (K)/5, Calculate Humidity Change/3(Temperature 1)
  Inlet Pressure (bar) (1 atm)/1 -> Bar to Pascal/1, Product/2
  Gain/1 -> Math Function/1
  Compressor  Map/1(Corrected Air Flow) -> To Workspace12/1, Product2/1
  Product/1 -> To Workspace13/1, Compressor  Map/1(Pressure Ratio In)
  1 Pressure Ratio 2 Air Mass Flow Rate 3 Efficiency 4 Speed (rad/sec) 5 Inlet Temp (K)/1 -> Change in Temperature/1, Power equation/1
  Pascal to Bar/1 -> Product/1
  Change in Temperature/1 -> Sum/1
  Divided by Mech eff/1 -> Power/1
  Power equation/1 -> Divided by Mech eff/1
  Compressor  Map/3(Pressure Ratio Out) -> 1 Pressure Ratio 2 Air Mass Flow Rate 3 Efficiency 4 Speed (rad/sec) 5 Inlet Temp (K)/1
  Gain1/1 -> Product2/2
  Math Function/1 -> Product2/3, Product1/2
  Ambient Pressure (atm)/1 -> Gain1/1
  Ambient Air Temp (K)/1 -> Gain/1
  rad/sec to rpm/1 -> Product1/1
  Product1/1 -> Compressor  Map/2(Corrected Speed (rpm))
  Compressor  Map/2(Efficiency) -> 1 Pressure Ratio 2 Air Mass Flow Rate 3 Efficiency 4 Speed (rad/sec) 5 Inlet Temp (K)/3
  Speed/1 -> 1 Pressure Ratio 2 Air Mass Flow Rate 3 Efficiency 4 Speed (rad/sec) 5 Inlet Temp (K)/4, rad/sec to rpm/1
  Product2/1 -> 1 Pressure Ratio 2 Air Mass Flow Rate 3 Efficiency 4 Speed (rad/sec) 5 Inlet Temp (K)/2, To Workspace1/1, 1 - Total Mass Flow 2 - Temperature 3 - Pressure 4 - Relative Humidity 5 - Oxygen Mole Fraction (in Dry Air)1/1
  Exit Pressure (Pa)/1 -> Calculate Humidity Change/2(Pressure 2), Pascal to Bar/1, 1 - Total Mass Flow 2 - Temperature 3 - Pressure 4 - Relative Humidity 5 - Oxygen Mole Fraction (in Dry Air)1/3
  1 - Total Mass Flow 2 - Temperature 3 - Pressure 4 - Relative Humidity 5 - Oxygen Mole Fraction (in Dry Air)1/1 -> CP Flow/1

== system fcsystemBechmarkold/Fuel Cell Stack System/Compressor/Static Motor ==
  Input Voltage : Inport
  Motor Speed (rad/s) : Inport  Port=2
  1/R : Gain  Gain=1/cm_R  SaturateOnIntegerOverflow=on  OutDataTypeStr=Inherit: Same as input  ParamDataTypeStr=Inherit: Same as input
  Constant : Constant  Value=cm_kv
  Electrical Efficiency : Display
  Mech Eff. : Gain  SaturateOnIntegerOverflow=on  OutDataTypeStr=Inherit: Same as input  ParamDataTypeStr=Inherit: Same as input
  Product : Product  SaturateOnIntegerOverflow=on  InputSameDT=on  OutDataTypeStr=Inherit: Same as first input
  Product1 : Product  SaturateOnIntegerOverflow=on  InputSameDT=on  OutDataTypeStr=Inherit: Same as first input
  Product2 : Product  SaturateOnIntegerOverflow=on  InputSameDT=on  OutDataTypeStr=Inherit: Same as first input
  Product3 : Product  Inputs=/*  SaturateOnIntegerOverflow=on  InputSameDT=on  OutDataTypeStr=Inherit: Same as first input
  Saturation : Saturate  UpperLimit=cm_maxtorque  LowerLimit=-cm_maxtorque
  Sum : Sum  Inputs=+-  SaturateOnIntegerOverflow=on  InputSameDT=on  OutDataTypeStr=Inherit: Same as first input
  To Workspace1 : ToWorkspace  VariableName=outCMtorque  SampleTime=-1
  kt : Gain  Gain=cm_kt  SaturateOnIntegerOverflow=on  OutDataTypeStr=Inherit: Same as input  ParamDataTypeStr=Inherit: Same as input
  Motor Power : Outport
  Motor Current : Outport  Port=2
  wires:
  Product3/1 -> Electrical Efficiency/1
  Product2/1 -> Product3/2, Mech Eff./1
  Product1/1 -> Product3/1
  Input Voltage/1 -> Product2/1, Sum/1
  1/R/1 -> Motor Current/1, Product2/2, kt/1
  kt/1 -> Saturation/1
  Saturation/1 -> Product1/1, To Workspace1/1
  Sum/1 -> 1/R/1
  Product/1 -> Sum/2
  Constant/1 -> Product/1
  Motor Speed (rad/s)/1 -> Product/2, Product1/2
  Mech Eff./1 -> Motor Power/1

== system fcsystemBechmarkold/Fuel Cell Stack System/Compressor/Turbocharger Inertia ==
  Motor Power : Inport
  Compressor Power : Inport  Port=2
  Turbine Power : Inport  Port=3
  Compressor speed : Integrator  InitialConditionSource=external  InitialCondition=10069.57894
  Divided by Inertia : Gain  Gain=1/cp_inertia  SaturateOnIntegerOverflow=on  OutDataTypeStr=Inherit: Same as input  ParamDataTypeStr=Inherit: Same as input
  IC : Constant  Value=fcx0(4)
  Product1 : Product  Inputs=*/  SaturateOnIntegerOverflow=on  InputSameDT=on  OutDataTypeStr=Inherit: Same as first input
  Sum : Sum  Inputs=+-+  SaturateOnIntegerOverflow=on  InputSameDT=on  OutDataTypeStr=Inherit: Same as first input
  Speed : Outport
  tag scope: w_cp=global
  wires:
  Compressor speed/1 -> Speed/1, Product1/2, [w_cp]
  IC/1 -> Compressor speed/2
  Divided by Inertia/1 -> Compressor speed/1
  Turbine Power/1 -> Sum/3
  Compressor Power/1 -> Sum/2
  Motor Power/1 -> Sum/1
  Sum/1 -> Product1/1
  Product1/1 -> Divided by Inertia/1

== system fcsystemBechmarkold/Fuel Cell Stack System/Inlet Manifold/Calculate Humidity Change ==
  note: Pv2 = (P2/P1)*Pv1
      | Pa2 = (P2/P1)*Pa1
      | phi2 = Pv2/Psat(T2) = P2*Pv1/P1/Psat(T2) = P2*phi1*Psat(T1)/P1/Psat(T2)
  Pressure 1 : Inport
  Pressure 2 : Inport  Port=2
  Temperature 1 : Inport  Port=3
  Temperature 2 : Inport  Port=4
  Humidity 1 : Inport  Port=5
  Product : Product  Inputs=***//  SaturateOnIntegerOverflow=on  InputSameDT=on  OutDataTypeStr=Inherit: Same as first input
  Saturation 0-1 : Saturate  UpperLimit=1  LowerLimit=0
  Saturation Pressure (Pa) : Subsystem
  Saturation Pressure (Pa)1 : Subsystem
  Humidity 2 : Outport
  wires:
  Temperature 2/1 -> Saturation Pressure (Pa)1/1(Temperature (K))
  Humidity 1/1 -> Product/2
  Pressure 2/1 -> Product/1
  Pressure 1/1 -> Product/4
  Temperature 1/1 -> Saturation Pressure (Pa)/1(Temperature (K))
  Saturation Pressure (Pa)1/1(Saturation Pressure (Pa)) -> Product/5
  Saturation Pressure (Pa)/1(Saturation Pressure (Pa)) -> Product/3
  Product/1 -> Saturation 0-1/1
  Saturation 0-1/1 -> Humidity 2/1

== system fcsystemBechmarkold/Fuel Cell Stack System/Magic Cooler/Calculate Humidity Change ==
  note: Pv2 = (P2/P1)*Pv1
      | Pa2 = (P2/P1)*Pa1
      | phi2 = Pv2/Psat(T2) = P2*Pv1/P1/Psat(T2) = P2*phi1*Psat(T1)/P1/Psat(T2)
  Pressure 1 : Inport
  Pressure 2 : Inport  Port=2
  Temperature 1 : Inport  Port=3
  Temperature 2 : Inport  Port=4
  Humidity 1 : Inport  Port=5
  Display{,1..3} (4 alike) : Display
  Product : Product  Inputs=***//  SaturateOnIntegerOverflow=on  InputSameDT=on  OutDataTypeStr=Inherit: Same as first input
  Saturation 0-1 : Saturate  UpperLimit=1  LowerLimit=0
  Saturation Pressure (Pa) : Subsystem
  Saturation Pressure (Pa)1 : Subsystem
  Humidity 2 : Outport
  wires:
  Temperature 2/1 -> Saturation Pressure (Pa)1/1(Temperature (K))
  Humidity 1/1 -> Product/2
  Pressure 2/1 -> Product/1
  Pressure 1/1 -> Product/4
  Temperature 1/1 -> Saturation Pressure (Pa)/1(Temperature (K))
  Saturation Pressure (Pa)1/1(Saturation Pressure (Pa)) -> Product/5, Display/1
  Saturation Pressure (Pa)/1(Saturation Pressure (Pa)) -> Product/3, Display1/1
  Product/1 -> Display2/1, Saturation 0-1/1
  Saturation 0-1/1 -> Humidity 2/1, Display3/1

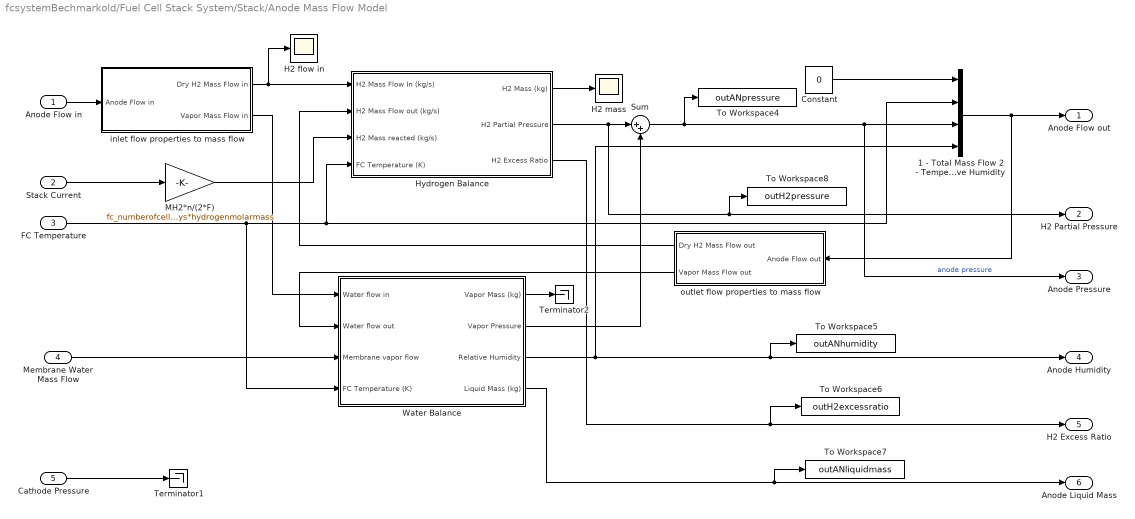
== system fcsystemBechmarkold/Fuel Cell Stack System/Stack/Anode Mass Flow Model ==
  Anode Flow in : Inport
  Stack Current : Inport  Port=2
  FC Temperature : Inport  Port=3
  Membrane Water Mass Flow : Inport  Port=4
  Cathode Pressure : Inport  Port=5
  1 - Total Mass Flow 2 - Temperature 3 - Pressure 4 - Relative Humidity : Mux
  Constant : Constant  Value=0
  H2 flow in : Scope
  H2 mass : Scope
  Hydrogen Balance : Subsystem
  MH2*n/(2*F) : Gain  Gain=fc_numberofcells/2/faradays*hydrogenmolarmass  SaturateOnIntegerOverflow=on  OutDataTypeStr=Inherit: Same as input  ParamDataTypeStr=Inherit: Same as input
  Sum : Sum  Inputs=|++  SaturateOnIntegerOverflow=on  InputSameDT=on  OutDataTypeStr=Inherit: Same as first input
  Terminator1 : Terminator
  Terminator2 : Terminator
  To Workspace4 : ToWorkspace  VariableName=outANpressure  SampleTime=-1
  To Workspace5 : ToWorkspace  VariableName=outANhumidity  SampleTime=-1
  To Workspace6 : ToWorkspace  VariableName=outH2excessratio  SampleTime=-1
  To Workspace7 : ToWorkspace  VariableName=outANliquidmass  SampleTime=-1
  To Workspace8 : ToWorkspace  VariableName=outH2pressure  SampleTime=-1
  Water Balance : Subsystem
  inlet flow properties to mass flow : Subsystem
  outlet flow properties to mass flow : Subsystem
  Anode Flow out : Outport
  H2 Partial Pressure : Outport  Port=2
  Anode Pressure : Outport  Port=3
  Anode Humidity : Outport  Port=4
  H2 Excess Ratio : Outport  Port=5
  Anode Liquid Mass : Outport  Port=6
  wires:
  Hydrogen Balance/1(H2 Mass (kg)) -> H2 mass/1
  Hydrogen Balance/2(H2 Partial Pressure) -> To Workspace8/1, H2 Partial Pressure/1, Sum/1
  MH2*n/(2*F)/1 -> Hydrogen Balance/3(H2 Mass reacted (kg/s))
  Water Balance/4(Liquid Mass (kg)) -> To Workspace7/1, Anode Liquid Mass/1
  Hydrogen Balance/3(H2 Excess Ratio) -> H2 Excess Ratio/1, To Workspace6/1
  Sum/1 -> To Workspace4/1, Anode Pressure/1, 1 - Total Mass Flow 2 - Temperature 3 - Pressure 4 - Relative Humidity/3  "anode pressure"
  outlet flow properties to mass flow/2(Vapor Mass Flow out) -> Water Balance/2(Water flow out)
  Membrane Water Mass Flow/1 -> Water Balance/3(Membrane vapor flow)
  FC Temperature/1 -> Water Balance/4(FC Temperature (K)), 1 - Total Mass Flow 2 - Temperature 3 - Pressure 4 - Relative Humidity/2, Hydrogen Balance/4(FC Temperature (K))
  1 - Total Mass Flow 2 - Temperature 3 - Pressure 4 - Relative Humidity/1 -> outlet flow properties to mass flow/1(Anode Flow out), Anode Flow out/1
  Anode Flow in/1 -> inlet flow properties to mass flow/1(Anode Flow in)
  outlet flow properties to mass flow/1(Dry H2 Mass Flow out) -> Hydrogen Balance/2(H2 Mass Flow out (kg/s))
  inlet flow properties to mass flow/1(Dry H2 Mass Flow in) -> Hydrogen Balance/1(H2 Mass Flow In (kg/s)), H2 flow in/1
  inlet flow properties to mass flow/2(Vapor Mass Flow in) -> Water Balance/1(Water flow in)
  Water Balance/3(Relative Humidity) -> To Workspace5/1, Anode Humidity/1, 1 - Total Mass Flow 2 - Temperature 3 - Pressure 4 - Relative Humidity/4
  Water Balance/2(Vapor Pressure) -> Sum/2
  Water Balance/1(Vapor Mass (kg)) -> Terminator2/1
  Stack Current/1 -> MH2*n/(2*F)/1
  Cathode Pressure/1 -> Terminator1/1
  Constant/1 -> 1 - Total Mass Flow 2 - Temperature 3 - Pressure 4 - Relative Humidity/1
